simulink model "Obstacles"  (R2021a)
settings: Solver=VariableStepAuto  StartTime=0.0  StopTime=1  RelTol=1e-3
values from neighbouring files (symbols this model uses):
  obst = [[-5183,-1720];[-3948,-2387];[0,1080];[-3513,-2868];[2500,3100];[-3259,-3303];[-3323,-4296];[-3948,-3598];[-4996,-3466];[-4581,-2868]]    [path_obst.m]
undefined symbols (not defined in the file or in its folder): L

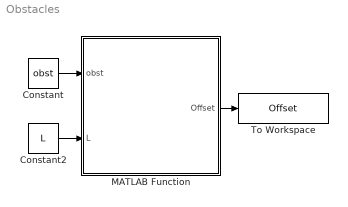
== system Obstacles ==
  Constant : Constant  Value=obst
  Constant2 : Constant  Value=L
  MATLAB Function : MATLAB Function  TreatAsAtomicUnit=on
  To Workspace : ToWorkspace  VariableName=Offset  SampleTime=1
  wires:
  Constant/1 -> MATLAB Function/1(obst)
  Constant2/1 -> MATLAB Function/2(L)
  MATLAB Function/1(Offset) -> To Workspace/1

== matlab function Obstacles/MATLAB Function ==
function Offset = fcn(obst,L)
L=-L;
Offset=zeros(size(obst));
a=size(obst);
N=a(1);
for i=1:N
    if i>1
    pre = i-1;
    else 
      pre = N; 
    end
    if i<N
     post = i+1;
    else 
      post = 1; 
    end
X1=((obst(i,1)-obst(pre,1))/sqrt((obst(i,1)-obst(pre,1))^2+((obst(i,2)-obst(pre,2)))^2));
X2=((obst(i,1)-obst(post,1))/sqrt((obst(i,1)-obst(post,1))^2+((obst(i,2)-obst(post,2)))^2));
Y1=((obst(i,2)-obst(pre,2))/sqrt((obst(i,1)-obst(pre,1))^2+((obst(i,2)-obst(pre,2)))^2));
Y2=((obst(i,2)-obst(post,2))/sqrt((obst(i,1)-obst(post,1))^2+((obst(i,2)-obst(post,2)))^2));
sine=(X1*Y2-X2*Y1)/sqrt(X1^2+Y1^2)*sqrt(X2^2+Y2^2);
Offset(i,1)=obst(i,1)+L*(X1+X2)/abs(sine);
Offset(i,2)=obst(i,2)+L*(Y1+Y2)/abs(sine);
if i>1
  check =(obst(i,1)-obst(pre,1))*(Offset(i,2)-Offset(pre,2))-(obst(i,2)-obst(pre,2))*(Offset(i,1)-Offset(pre,1)); 
 if abs(check) > 0.5
      Offset(i,1)=obst(i,1)-L*(X1+X2)/abs(sine);
      Offset(i,2)=obst(i,2)-L*(Y1+Y2)/abs(sine);
 end
end
end
